simulink model "onlyProportional"  (R2024b)
settings: Solver=VariableStepAuto  StartTime=0  StopTime=15  FixedStep=0.001  RelTol=1e-3
InitFcn:
  | LCS_parameters
undefined symbols (not defined in the file or in its folder): gearRatio
libraries: simulink x2, Solver_SF x1
settings Model: Creator=account  LastModifiedBy=xoxi.1

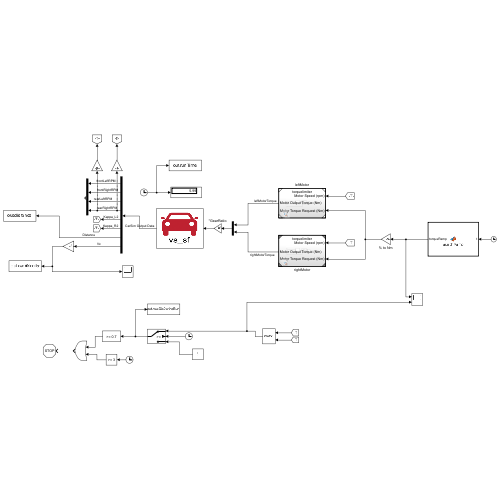
[thumbnail: Simulink's stored preview of the top-level diagram]
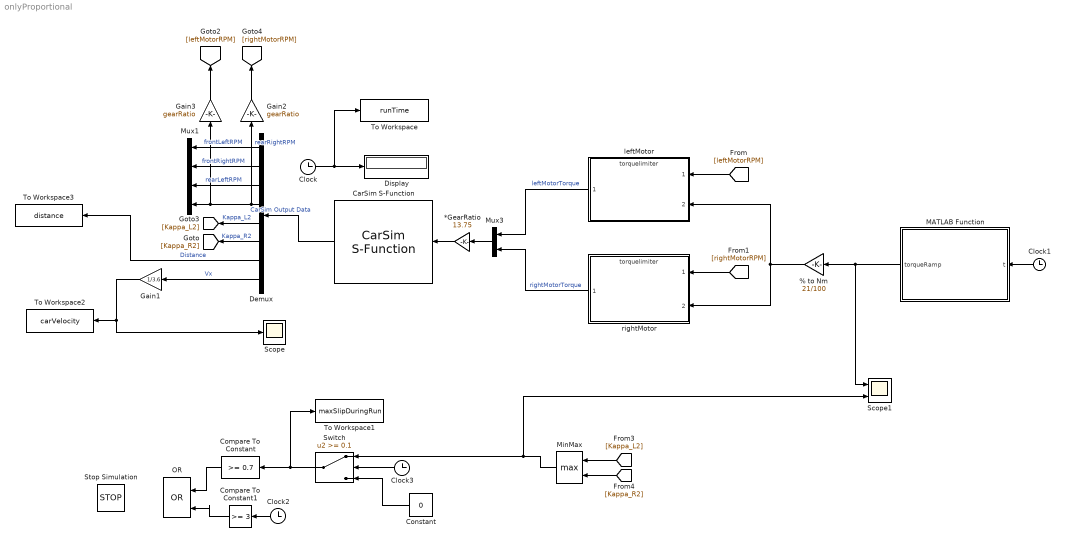
== system onlyProportional ==
  % to Nm : Gain  Gain=21/100
  *GearRatio : Gain  Gain=13.75
  CarSim S-Function : Solver_SF/CarSim S-Function  Priority=1  SIMFILE=simfile.sim  Run_RTs=off  vs_state_ind=Run  StopMode_ind=Vehicle Model
  Clock{,1..3} (4 alike) : Clock
  Compare To Constant : simulink/Logic and Bit Operations/Compare To Constant  relop=>=  const=0.7  OutDataTypeStr=boolean
  Compare To Constant1 : simulink/Logic and Bit Operations/Compare To Constant  relop=>=  const=3  OutDataTypeStr=boolean
  Constant : Constant  Value=0
  Demux : Demux  Outputs=8
  Display : Display
  Gain1 : Gain  Gain=1/3.6
  Gain2 : Gain  Gain=gearRatio
  Gain3 : Gain  Gain=gearRatio
  MATLAB Function : MATLAB Function  TreatAsAtomicUnit=on
  MinMax : MinMax  Function=max  Inputs=2
  Mux1 : Mux
  Mux3 : Mux  Inputs=2
  OR : Logic  Operator=OR  IconShape=distinctive  AllPortsSameDT=off  OutDataTypeStr=boolean
  Scope : Scope
  Scope1 : Scope  NumInputPorts=2
  Stop Simulation : Stop
  Switch : Switch  Threshold=0.1  SaturateOnIntegerOverflow=off  InputSameDT=off
  To Workspace : ToWorkspace  VariableName=runTime  SaveFormat=Timeseries  SampleTime=-1
      settings: Save2DSignal=2-D array (concatenate along first dimension)
  To Workspace1 : ToWorkspace  VariableName=maxSlipDuringRun  SampleTime=-1
      settings: Save2DSignal=2-D array (concatenate along first dimension)
  To Workspace2 : ToWorkspace  VariableName=carVelocity  SampleTime=-1
      settings: Save2DSignal=2-D array (concatenate along first dimension)
  To Workspace3 : ToWorkspace  VariableName=distance  SampleTime=-1
      settings: Save2DSignal=2-D array (concatenate along first dimension)
  leftMotor : ModelReference  ModelNameDialog=torquelimiter.slx  SimulationMode=Normal  ModelReferenceVersion=1.5
  rightMotor : ModelReference  ModelNameDialog=torquelimiter.slx  SimulationMode=Normal  ModelReferenceVersion=1.5
  wires:
  CarSim S-Function/1 -> Demux/1  "CarSim Output Data"
  Demux/1 -> Mux1/1  "frontLeftRPM"
  Demux/2 -> Mux1/2  "frontRightRPM"
  Demux/3 -> Mux1/3  "rearLeftRPM"
  Clock/1 -> To Workspace/1, Display/1
  leftMotor/1 -> Mux3/1  "leftMotorTorque"
  rightMotor/1 -> Mux3/2  "rightMotorTorque"
  Demux/4 -> Mux1/4, Gain3/1, Gain2/1  "rearRightRPM"
  [rightMotorRPM] -> rightMotor/1
  [leftMotorRPM] -> leftMotor/1
  Demux/5 -> [Kappa_L2]  "Kappa_L2"
  Demux/6 -> [Kappa_R2]  "Kappa_R2"
  % to Nm/1 -> leftMotor/2, rightMotor/2
  *GearRatio/1 -> CarSim S-Function/1
  Mux3/1 -> *GearRatio/1
  Gain3/1 -> [leftMotorRPM]
  Gain2/1 -> [rightMotorRPM]
  Gain1/1 -> Scope/1, To Workspace2/1
  MinMax/1 -> Scope1/2, Switch/1
  [Kappa_L2] -> MinMax/1
  [Kappa_R2] -> MinMax/2
  Compare To Constant1/1 -> OR/2
  Clock2/1 -> Compare To Constant1/1
  Compare To Constant/1 -> OR/1
  Demux/8 -> Gain1/1  "Vx"
  Demux/7 -> To Workspace3/1  "Distance"
  Clock1/1 -> MATLAB Function/1(t)
  MATLAB Function/1(torqueRamp) -> Scope1/1, % to Nm/1
  Switch/1 -> To Workspace1/1, Compare To Constant/1
  Clock3/1 -> Switch/2
  Constant/1 -> Switch/3

== matlab function onlyProportional/MATLAB Function ==
  data: t input; torqueRamp output
function torqueRamp = launchRamp(t)
  if t <= 1.0
      torqueRamp = -295.875*t^4 + 816.75*t^3 - 798.125*t^2 + 329.5*t + 33.75;
elseif t <= 2.0
      s = t - 1.0;
      torqueRamp = -1.185185185*s^4 + (-14.81481481)*s^3 + 28.51851852*s^2 + (-3.518518519)*s + 86;
elseif t <= 2.4
      s = t - 2.0;
      torqueRamp = -156.25*s^3 + 93.75*s^2 + 95;
else
      torqueRamp = 100;
end
  torqueRamp = min(max(torqueRamp, 0), 100);
end
